simulink model "inverted_pendulum_fc"  (R2024a)
settings: Solver=VariableStepAuto  StartTime=0  StopTime=10  FixedStep=0.02  MaxStep=0.02  RelTol=1e-3  AbsTol=1e-6
libraries: fuzblock x1
CloseFcn:
  | set(groot,'ShowHiddenHandles','on');
  | c = get(groot,'Children');
  | close(c);
  | clear c;
  | set(groot,'ShowHiddenHandles','off');
Description:
  | Inverted Pendulum with Animation
  | 
  | This example shows how to model an inverted pendulum.  The animation is created using MATLAB(R) Handle Graphics(R).  The animation block is a masked
  | S-function.  For more information, use the context menu to look under the Animation block's mask
  | and open the S-function for editing.
settings Model: Creator=The MathWorks, Inc.  LastModifiedBy=wangb
settings SolverCC: AutoScaleAbsTol=off  AlgebraicLoopSolver=TrustRegion
settings DataIOCC: ExternalInput=[]  InitialState=[]  SaveFormat=Array  SaveOutput=off  SaveTime=off
settings OptimizationCC: BlockReduction=off  BooleanDataType=off  ReuseModelBlockBuffer=off  ExpressionDepthLimit=2147483647  InitFltsAndDblsToZero=on  LifeSpan=inf
settings DebuggingCC: SaveWithParameterizedLinksMsg=none  UnderspecifiedInitializationDetection=Classic  MergeDetectMultiDrivingBlocksExec=none  SignalResolutionControl=TryResolveAllWithWarning  MultiTaskDSMMsg=warning  MultiTaskCondExecSysMsg=none  SigSpecEnsureSampleTimeMsg=none  FcnCallInpInsideContextMsg=warning  UnconnectedInputMsg=warning  UnconnectedOutputMsg=warning  UnconnectedLineMsg=warning  StateNameClashWarn=warning  SubsystemReferenceDiagnosticForUnitTest=warning  SFUnexpectedBacktrackingDiag=warning  SFNoUnconditionalDefaultTransitionDiag=warning  SFExecutionAtInitializationDiag=none  ArithmeticOperatorsInVariantConditions=warning
settings HardwareCC: ProdBitPerPointer=32  ProdBitPerSizeT=32  ProdBitPerPtrDiffT=32  ProdLargestAtomicFloat=None  ProdIntDivRoundTo=Undefined  ProdEndianess=Unspecified  ProdWordSize=32  ProdHWDeviceType=32-bit Generic  TargetUnknown=on
settings ModelReferenceCC: EnableRefExpFcnMdlSchedulingChecks=on  PropagateSignalLabelsOutOfModel=off
settings SFSimCC: SimUseLocalCustomCode=off  CustomCodeUndefinedFunction=UseInterfaceOnly
settings RTWCC: RTWUseLocalCustomCode=off  GPUComputeCapability=3.5
settings CodeAppCC: StateflowObjectComments=on
settings GRTTargetCC: TargetFcnLib=ansi_tfl_tmw.mat  TargetLangStandard=C89/C90 (ANSI)  CombineOutputUpdateFcns=off  GRTInterface=on
settings ConfigComp: CovMetricSettings=dw  CovSaveCumulativeToWorkspaceVar=on  CovSaveSingleToWorkspaceVar=on  CovExternalEMLEnable=off

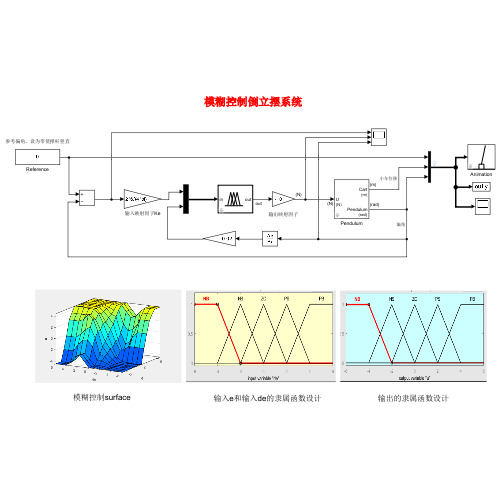
[thumbnail: Simulink's stored preview of the top-level diagram]
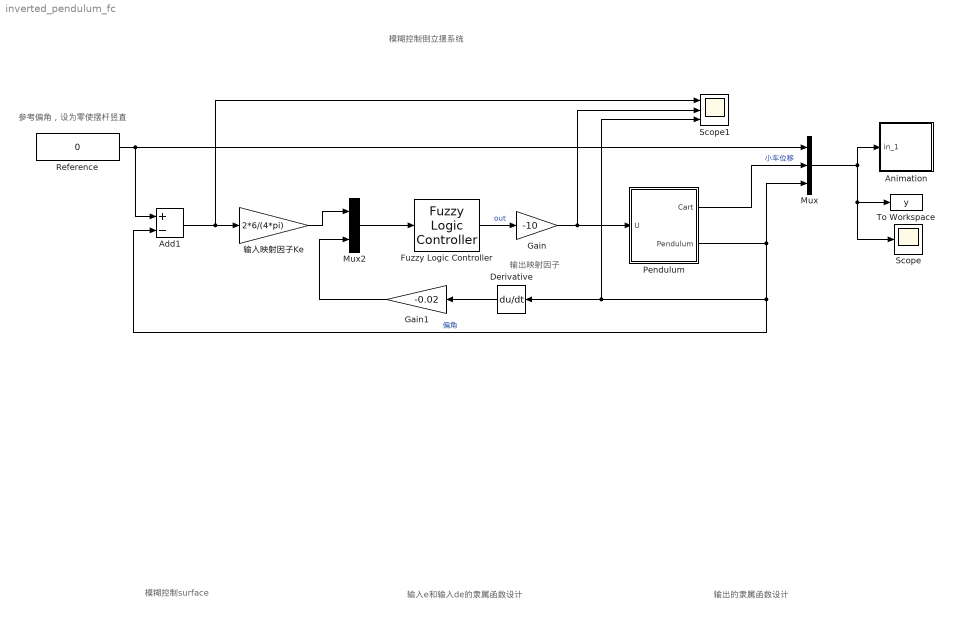
== system inverted_pendulum_fc ==
  note: 参考偏角，设为零使摆杆竖直
  note: 模糊控制surface
  note: 模糊控制倒立摆系统
  note: 输出映射因子
  note: 输出的隶属函数设计
  note: 输入e和输入de的隶属函数设计
  Add1 : Sum  Inputs=+-
  Animation : Subsystem  mask(Pendulum plot){RefBlock=Reference}
      mask prompts: RefBlock "DC reference signal block name:"
      mask help: Pendulum plot
      mask Help: Pendulum animation function using Handle graphics.
      mask Display: plot([-10 10],[0 0],[-2 -2 2 2],[0 1 1 0],[0 3],[1 5])
  Derivative : Derivative
  Fuzzy Logic Controller : fuzblock/Fuzzy Logic  Controller  FIS=fuzzy_control  OutputSampleNumber=101  DataType=double  FuzzifiedInputs=off  RuleFiringStrengths=off  RuleOutputs=off  AggregatedOutputs=off  SimulateUsing=Interpreted execution  OutOfRangeInputValueMessage=warning  NoRuleFiredMessage=warning  EmptyOutputFuzzySetMessage=warning
  Gain : Gain  Gain=-10
  Gain1 : Gain  Gain=-0.02
  Mux : Mux  Inputs=3
  Mux2 : Mux  Inputs=2
  Pendulum : Subsystem  mask(Inverted Pendulum Dynamics){Mcart=0.455, m=0.21, l=0.61/2, g=9.8}
      mask prompts: Mcart "Mass of cart (kg):"; m "Mass of pendulum (kg):"; l "Distance to pendulum center of mass (m):"; g "Acceleration of gravity (m/s^2):"
      mask help: Masked subsystem containing nonlinear dynamics of inverted pendulum on a cart.
      mask Help: Nonlinear dynamics of inverted pendulum on cart.
  Reference : Constant  Value=0
  Scope : Scope
  Scope1 : Scope  NumInputPorts=3
  To Workspace : ToWorkspace  VariableName=y  SampleTime=0.1
  输入映射因子Ke : Gain  Gain=2*6/(4*pi)
  wires:
  Mux/1 -> Scope/1, To Workspace/1, Animation/1(in_1)
  Pendulum/1(Cart) -> Mux/2  "小车位移"
  Reference/1 -> Add1/1, Mux/1
  Pendulum/2(Pendulum) -> Mux/3, Scope1/3, Derivative/1, Add1/2  "偏角"
  Gain/1 -> Pendulum/1(U), Scope1/2
  Fuzzy Logic Controller/1 -> Gain/1  "out"
  Derivative/1 -> Gain1/1
  Add1/1 -> 输入映射因子Ke/1, Scope1/1
  Mux2/1 -> Fuzzy Logic Controller/1
  输入映射因子Ke/1 -> Mux2/1
  Gain1/1 -> Mux2/2

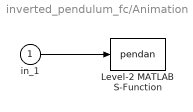
== system inverted_pendulum_fc/Animation ==
  in_1 : Inport
  Level-2 MATLAB S-Function : M-S-Function  FunctionName=pendan  Parameters=RefBlock
  wires:
  in_1/1 -> Level-2 MATLAB S-Function/1

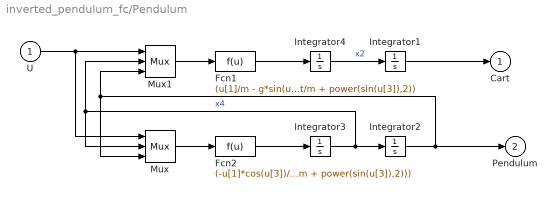
== system inverted_pendulum_fc/Pendulum ==
  U : Inport  Unit=N
  Fcn1 : Fcn  Expr=(u[1]/m - g*sin(u[3])*cos(u[3]) + l*power(u[2],2)*sin(u[3]))/(Mcart/m + power(sin(u[3]),2))
  Fcn2 : Fcn  Expr=(-u[1]*cos(u[3])/m + (Mcart+m)*g*sin(u[3])/m - l*power(u[2],2)*sin(u[3])*cos(u[3]))/(l*(Mcart/m + power(sin(u[3]),2)))
  Integrator1 : Integrator
  Integrator2 : Integrator  InitialCondition=0.3
  Integrator3 : Integrator
  Integrator4 : Integrator
  Mux : Mux  Inputs=3
  Mux1 : Mux  Inputs=3
  Cart : Outport  Unit=m  InitialOutput=0  VectorParamsAs1DForOutWhenUnconnected=off
  Pendulum : Outport  Port=2  Unit=rad  InitialOutput=0  VectorParamsAs1DForOutWhenUnconnected=off
  wires:
  Integrator1/1 -> Cart/1
  Fcn2/1 -> Integrator3/1
  Mux/1 -> Fcn2/1
  Mux1/1 -> Fcn1/1
  Fcn1/1 -> Integrator4/1
  Integrator4/1 -> Integrator1/1  "x2"
  U/1 -> Mux1/1, Mux/1
  Integrator3/1 -> Integrator2/1, Mux1/2, Mux/2  "x4"
  Integrator2/1 -> Pendulum/1, Mux1/3, Mux/3
